simulink model "Model_3D_NL"  (R2016b)
settings: Solver=FixedStepAuto  StartTime=0.0  StopTime=10.0  FixedStep=0.001  RelTol=1e-3
undefined symbols (not defined in the file): C_psi, I_K_inv, I_R_inv, Kd, l_C, m, T_Kd, T_red, Ta, x_0
libraries: vrlib x2
settings Model: Creator=michael  LastModifiedBy=michael

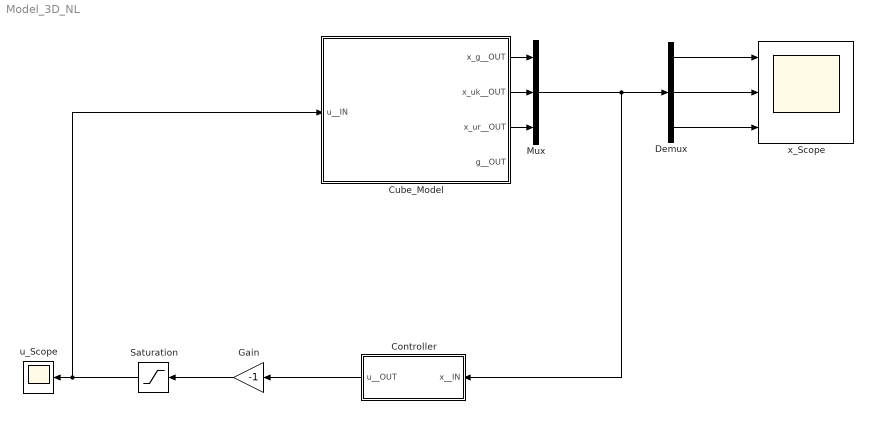
== system Model_3D_NL ==
  Controller : Subsystem
  Cube_Model : Subsystem
  Demux : Demux  Outputs=3
  Gain : Gain  Gain=-1
  Mux : Mux  Inputs=3
  Saturation : Saturate  UpperLimit=0.13  LowerLimit=-0.13
  u_Scope : Scope
  x_Scope : Scope  NumInputPorts=3
  wires:
  Controller/1(u__OUT) -> Gain/1
  Cube_Model/2(x_uk__OUT) -> Mux/2
  Cube_Model/1(x_g__OUT) -> Mux/1
  Cube_Model/3(x_ur__OUT) -> Mux/3
  Mux/1 -> Demux/1, Controller/1(x__IN)
  Gain/1 -> Saturation/1
  Demux/2 -> x_Scope/2
  Demux/1 -> x_Scope/1
  Demux/3 -> x_Scope/3
  Saturation/1 -> u_Scope/1, Cube_Model/1(u__IN)

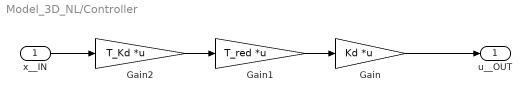
== system Model_3D_NL/Controller ==
  x__IN : Inport  SampleTime=Ta
  Gain : Gain  Gain=Kd  Multiplication=Matrix(K*u) (u vector)
  Gain1 : Gain  Gain=T_red  Multiplication=Matrix(K*u) (u vector)
  Gain2 : Gain  Gain=T_Kd  Multiplication=Matrix(K*u) (u vector)
  u__OUT : Outport
  wires:
  Gain/1 -> u__OUT/1
  Gain1/1 -> Gain/1
  Gain2/1 -> Gain1/1
  x__IN/1 -> Gain2/1

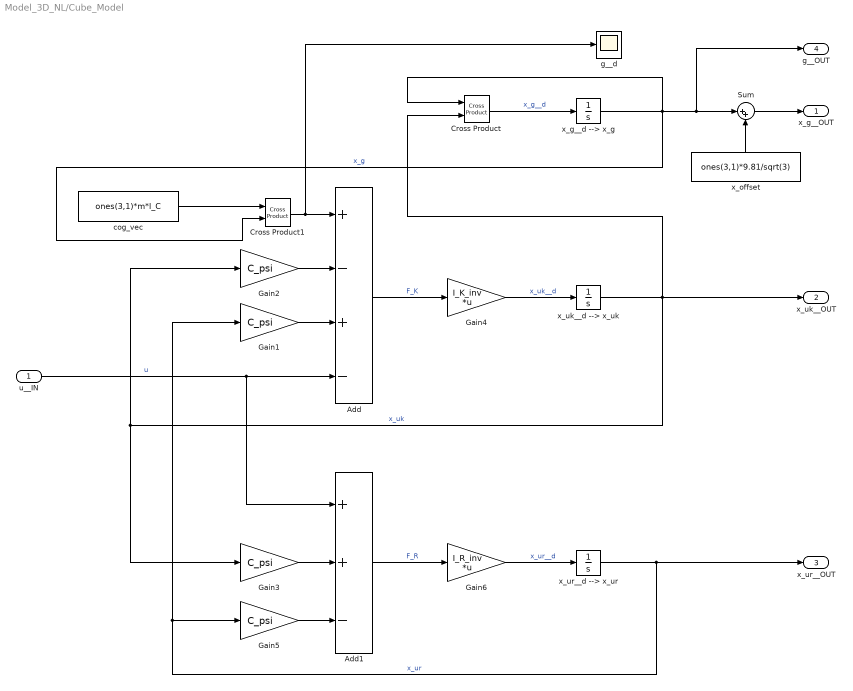
== system Model_3D_NL/Cube_Model ==
  u__IN : Inport
  Add : Sum  Inputs=+-+-
  Add1 : Sum  Inputs=++-
  Cross Product : vrlib/Utilities/Cross Product
  Cross Product1 : vrlib/Utilities/Cross Product
  Gain{1..3,5} (4 alike) : Gain  Gain=C_psi
  Gain4 : Gain  Gain=I_K_inv  Multiplication=Matrix(K*u) (u vector)
  Gain6 : Gain  Gain=I_R_inv  Multiplication=Matrix(K*u) (u vector)
  Sum : Sum  Inputs=|++
  cog_vec : Constant  Value=ones(3,1)*m*l_C
  g__d : Scope
  x_g__d --> x_g : Integrator  InitialCondition=x_0(1:3)
  x_offset : Constant  Value=ones(3,1)*9.81/sqrt(3)
  x_uk__d --> x_uk : Integrator  InitialCondition=x_0(4:6)
  x_ur__d --> x_ur : Integrator  InitialCondition=x_0(7:9)
  x_g__OUT : Outport
  x_uk__OUT : Outport  Port=2
  x_ur__OUT : Outport  Port=3
  g__OUT : Outport  Port=4
  wires:
  Add/1 -> Gain4/1  "F_K"
  Gain5/1 -> Add1/3
  Gain4/1 -> x_uk__d --> x_uk/1  "x_uk__d"
  Gain1/1 -> Add/3
  Gain2/1 -> Add/2
  u__IN/1 -> Add1/1, Add/4  "u"
  Gain3/1 -> Add1/2
  x_ur__d --> x_ur/1 -> x_ur__OUT/1, Gain1/1, Gain5/1  "x_ur"
  Gain6/1 -> x_ur__d --> x_ur/1  "x_ur__d"
  Add1/1 -> Gain6/1  "F_R"
  x_g__d --> x_g/1 -> Cross Product1/2, g__OUT/1, Sum/1, Cross Product/1  "x_g"
  x_uk__d --> x_uk/1 -> x_uk__OUT/1, Cross Product/2, Gain3/1, Gain2/1  "x_uk"
  Cross Product/1 -> x_g__d --> x_g/1  "x_g__d"
  Sum/1 -> x_g__OUT/1
  x_offset/1 -> Sum/2
  cog_vec/1 -> Cross Product1/1
  Cross Product1/1 -> g__d/1, Add/1
